simulink model "CRM_model_simulinkVersion"  (R2021b)
settings: Solver=VariableStepAuto  StartTime=0.0  StopTime=10.0  RelTol=1e-3
values from neighbouring files (symbols this model uses):
  C = 0.01    [CDM_testscript_transferFunctionApproach.m]
  R = 0.01    [CDM_testscript_transferFunctionApproach.m]
  X0 = 1    [CDM_testscript_transferFunctionApproach.m]
undefined symbols (not defined in the file or in its folder): c, d
settings Model: Creator=drkfr  LastModifiedBy=drkfr

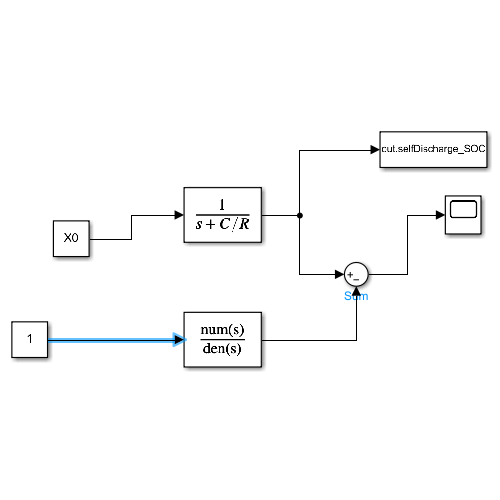
[thumbnail: Simulink's stored preview of the top-level diagram]
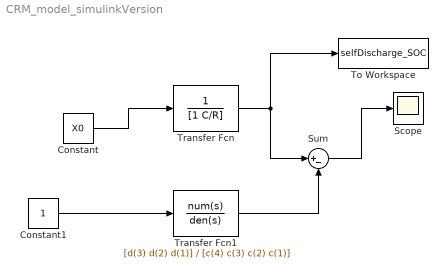
== system CRM_model_simulinkVersion ==
  Constant : Constant  Value=X0
  Constant1 : Constant
  Scope : Scope
  Sum : Sum  Inputs=|+-
  To Workspace : ToWorkspace  VariableName=selfDischarge_SOC  SaveFormat=Timeseries  SampleTime=-1
  Transfer Fcn : TransferFcn  Denominator=[1 C/R]
  Transfer Fcn1 : TransferFcn  Numerator=[d(3) d(2) d(1)]  Denominator=[c(4) c(3) c(2) c(1)]
  wires:
  Transfer Fcn/1 -> Sum/1, To Workspace/1
  Transfer Fcn1/1 -> Sum/2
  Sum/1 -> Scope/1
  Constant/1 -> Transfer Fcn/1
  Constant1/1 -> Transfer Fcn1/1
